simulink model "gm_FFTHDLOptimizedExample_Streaming"  (R2024a)
settings: Solver=FixedStepDiscrete  StartTime=0.0  StopTime=48*FFTLength/FrameSize  RelTol=1e-3
InitFcn:
  | FFTLength = 2^9;
  | Fs = 1*2e6;
  | FrameSize = 8;
  | ValidPattern = [1, 0];
libraries: dsphdlxfrm2 x1, dspmathops x1
settings Model: Creator=The MathWorks, Inc.  LastModifiedBy=Amir
settings SolverCC: AlgebraicLoopSolver=TrustRegion  MaxZcPerStep=1
settings DataIOCC: SaveOutput=off  SaveTime=off  ReturnWorkspaceOutputs=off
settings OptimizationCC: BlockReduction=off  ConditionallyExecuteInputs=off  DefaultParameterBehavior=Inlined
settings DebuggingCC: AlgebraicLoopMsg=error  InheritedTsInSrcMsg=none  SingleTaskRateTransMsg=error  UnconnectedInputMsg=warning  UnconnectedOutputMsg=warning  UnconnectedLineMsg=warning  ArithmeticOperatorsInVariantConditions=warning
settings HardwareCC: ProdBitPerPointer=32  ProdBitPerSizeT=32  ProdBitPerPtrDiffT=32  ProdLargestAtomicFloat=None  ProdIntDivRoundTo=Undefined  ProdEndianess=Unspecified  ProdWordSize=32  ProdHWDeviceType=ASIC/FPGA->ASIC/FPGA  ProdEqTarget=off
settings ModelReferenceCC: EnableRefExpFcnMdlSchedulingChecks=on
settings SFSimCC: SimUseLocalCustomCode=off  CustomCodeUndefinedFunction=UseInterfaceOnly
settings RTWCC: RTWUseLocalCustomCode=off  GPUComputeCapability=3.5  DLArmComputeVersion=19.05
settings CodeAppCC: StateflowObjectComments=on

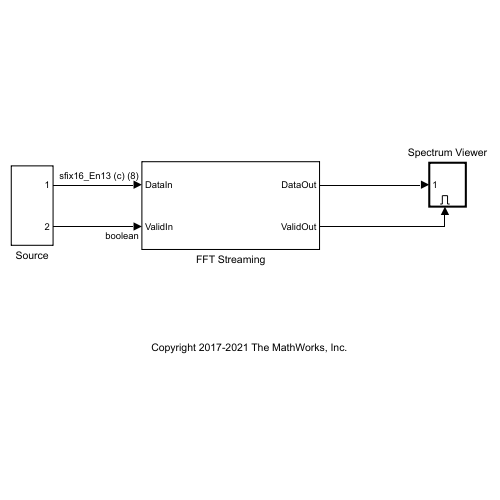
[thumbnail: Simulink's stored preview of the top-level diagram]
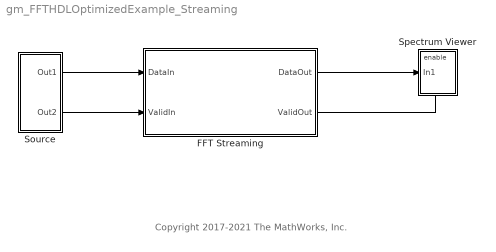
== system gm_FFTHDLOptimizedExample_Streaming ==
  note: Copyright 2017-2021 The MathWorks, Inc.
  FFT Streaming : Subsystem
  Source : Subsystem
  Spectrum Viewer : Subsystem
  wires:
  FFT Streaming/2(ValidOut) -> Spectrum Viewer/Enable
  Source/2(Out2) -> FFT Streaming/2(ValidIn)
  Source/1(Out1) -> FFT Streaming/1(DataIn)
  FFT Streaming/1(DataOut) -> Spectrum Viewer/1(In1)

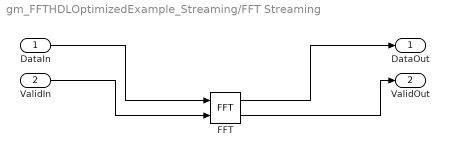
== system gm_FFTHDLOptimizedExample_Streaming/FFT Streaming ==
  DataIn : Inport  OutDataTypeStr=fixdt(1, 16, 13)  PortDimensions=[8]  SampleTime=1
      settings: SignalType=complex
  ValidIn : Inport  Port=2  OutDataTypeStr=boolean  PortDimensions=1  SampleTime=1
  FFT : dsphdlxfrm2/FFT  Architecture=Streaming Radix 2^2  FFTLengthSource=Property  FFTLength=FFTLength  FFTLengthMax=1024  ComplexMultiplication=Use 4 multipliers and 2 adders  BitReversedOutput=on  BitReversedInput=off  Normalize=off  SimulateUsing=Code generation  RoundingMethod=Floor  ResetInputPort=off  StartOutputPort=off  EndOutputPort=off
  DataOut : Outport  SampleTime=1  VectorParamsAs1DForOutWhenUnconnected=off
  ValidOut : Outport  Port=2  SampleTime=1  VectorParamsAs1DForOutWhenUnconnected=off
  wires:
  DataIn/1 -> FFT/1
  ValidIn/1 -> FFT/2
  FFT/1 -> DataOut/1
  FFT/2 -> ValidOut/1

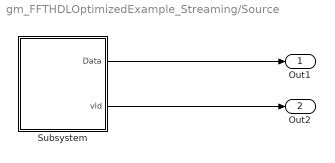
== system gm_FFTHDLOptimizedExample_Streaming/Source ==
  Subsystem : Subsystem
  Out1 : Outport  VectorParamsAs1DForOutWhenUnconnected=off
  Out2 : Outport  Port=2  VectorParamsAs1DForOutWhenUnconnected=off
  wires:
  Subsystem/1(Data) -> Out1/1
  Subsystem/2(vld) -> Out2/1

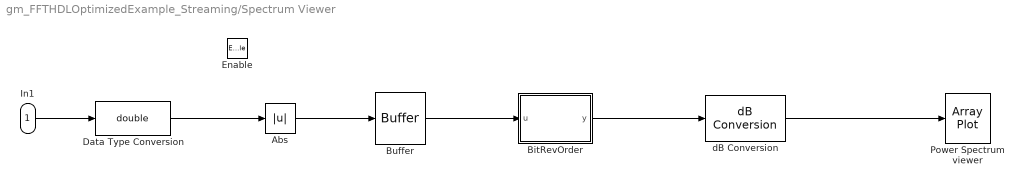
== system gm_FFTHDLOptimizedExample_Streaming/Spectrum Viewer ==
  In1 : Inport
  Enable : EnablePort
  Abs : Abs  SaturateOnIntegerOverflow=off
  BitRevOrder : MATLAB Function  TreatAsAtomicUnit=on
  Buffer : Buffer  N=FFTLength  OutputFrames=off
  Data Type Conversion : DataTypeConversion  OutDataTypeStr=double  SaturateOnIntegerOverflow=off  RndMeth=Floor
  Power Spectrum viewer : ArrayPlot  WindowPosition=[113.000000,151.000000,759.000000,428.000000,]  Visible=on  ScopeFrameLocation=window  SampleIncrement=Fs/FFTLength  PlotType=Stairs  AxesScaling=Manual  Title=Power Spectrum  XLabel=Frequency  YLabel=dBm  YLimits=[-60,60]  DefaultConfigurationName=dsp.scopes.ArrayPlotBlockSpecification
  dB Conversion : dspmathops/dB Conversion  dBtype=dB  intype=Amplitude  R=1  fuzz=on
  wires:
  In1/1 -> Data Type Conversion/1
  Abs/1 -> Buffer/1
  Data Type Conversion/1 -> Abs/1
  dB Conversion/1 -> Power Spectrum viewer/1
  BitRevOrder/1(y) -> dB Conversion/1
  Buffer/1 -> BitRevOrder/1(u)

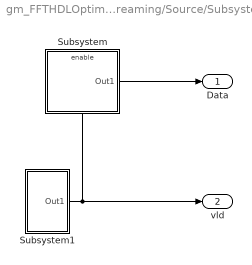
== system gm_FFTHDLOptimizedExample_Streaming/Source/Subsystem ==
  Subsystem : Subsystem
  Subsystem1 : Subsystem
  Data : Outport  VectorParamsAs1DForOutWhenUnconnected=off
  vld : Outport  Port=2  VectorParamsAs1DForOutWhenUnconnected=off
  wires:
  Subsystem/1(Out1) -> Data/1
  Subsystem1/1(Out1) -> Subsystem/Enable, vld/1

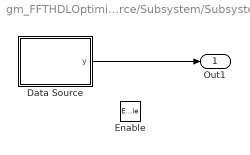
== system gm_FFTHDLOptimizedExample_Streaming/Source/Subsystem/Subsystem ==
  Enable : EnablePort
  Data Source : MATLAB Function  TreatAsAtomicUnit=on
  Out1 : Outport  VectorParamsAs1DForOutWhenUnconnected=off
  wires:
  Data Source/1(y) -> Out1/1

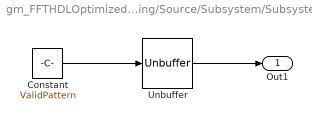
== system gm_FFTHDLOptimizedExample_Streaming/Source/Subsystem/Subsystem1 ==
  Constant : Constant  Value=ValidPattern  OutDataTypeStr=boolean  SampleTime=-1
  Unbuffer : Unbuffer
  Out1 : Outport  VectorParamsAs1DForOutWhenUnconnected=off
  wires:
  Unbuffer/1 -> Out1/1
  Constant/1 -> Unbuffer/1

== matlab function gm_FFTHDLOptimizedExample_Streaming/Source/Subsystem/Subsystem/Data Source ==
  settings: updateMethod=DISCRETE  sampleTime=1
  data: y output size=FrameSize; Fs parameter; FrameSize parameter
function y = fcn(Fs, FrameSize)
persistent sinegen1 sinegen2
noiseVar   = 1e-12;
if isempty(sinegen1)
    sinegen1 = dsp.SineWave('Amplitude', 1, 'Frequency',200000, 'SampleRate',Fs,'SamplesPerFrame',FrameSize);
    sinegen2 = dsp.SineWave('Amplitude', 2, 'Frequency',250000, 'SampleRate',Fs,'SamplesPerFrame',FrameSize); 
end

y = complex(fi(sinegen1() + sinegen2() + sqrt(noiseVar)*randn(FrameSize,1), 1, 16, 13));

== matlab function gm_FFTHDLOptimizedExample_Streaming/Spectrum Viewer/BitRevOrder ==
  data: u input; y output size=[FFTLength, 1]
function y = fcn(u)

%#codegen

y = bitrevorder(u);
